simulink model "PID_Tuning"  (R2016b)
settings: Solver=ode45  StartTime=0.0  StopTime=10.0  RelTol=1e-3  EnableMultiTasking=on
values from neighbouring files (symbols this model uses):
  dm = 3.8E-6    (= 3.8e-06)    [param.m]    (also in param_2.m)
  eps_dm = 1    [param.m]    (also in param_2.m)
  eps_Jeq = 1    [param.m]    (also in param_2.m)
  Jeq = Jm + (J1+J2)/(n^2)    (= 3.6746e-05)    [param.m]    (also in param_2.m)
  Kemf = 1/(137*2*pi/60)    (= 0.0697028947848)    [param.m]    (also in param_2.m)
  Km = 69.7E-3    (= 0.0697)    [param.m]    (also in param_2.m)
  n = 1    [param.m]    (also in param_2.m)
  R = 112    [param.m]    (also in param_2.m)
  Ts = 1e-2    (= 0.01)    [param.m]    (also in param_2.m = 0.001)
libraries: simulink x1
settings Model: Creator=diegogm  LastModifiedBy=diego
settings DataIOCC: LimitDataPoints=on
settings OptimizationCC: LifeSpan=inf
settings DebuggingCC: AllowSymbolicDim=off  SFUnexpectedBacktrackingDiag=warning  SFNoUnconditionalDefaultTransitionDiag=warning  SFExecutionAtInitializationDiag=none
settings ModelReferenceCC: PropagateSignalLabelsOutOfModel=off
settings GRTTargetCC: TargetLangStandard=C89/C90 (ANSI)
settings ConfigComp: CovMetricSettings=dw  CovHtmlReporting=on  CovSaveCumulativeToWorkspaceVar=on  CovSaveSingleToWorkspaceVar=on  CovExternalEMLEnable=off

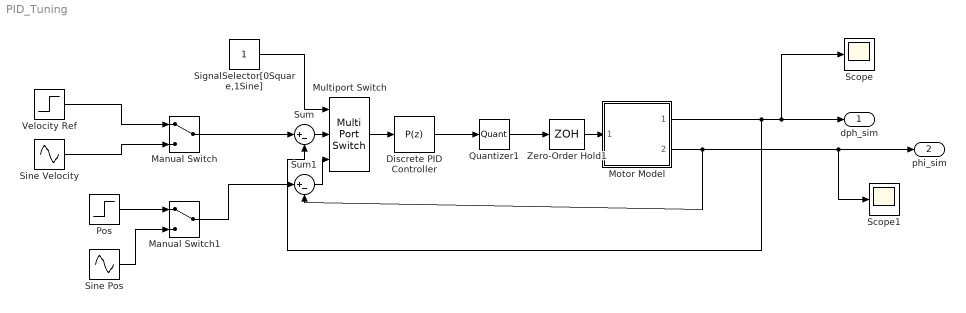
== system PID_Tuning ==
  Discrete PID Controller : simulink/Continuous/PID Controller  Controller=P  TimeDomain=Discrete-time  SampleTime=Ts  IntegratorMethod=Forward Euler  FilterMethod=Forward Euler  Form=Parallel  UseFilter=on  ControllerParametersSource=internal  P=1  I=1  D=1  N=1  InitialConditionSource=internal  InitialConditionForIntegrator=0  InitialConditionForFilter=0  ExternalReset=none  LimitOutput=off  UpperSaturationLimit=inf  LowerSaturationLimit=-inf  LinearizeAsGain=off  AntiWindupMode=none  Kb=1  TrackingMode=off  Kt=1  PParamMin=[]  PParamMax=[]  IParamMin=[]  IParamMax=[]  DParamMin=[]  DParamMax=[]  NParamMin=[]  NParamMax=[]  KbParamMin=[]  KbParamMax=[]  KtParamMin=[]  KtParamMax=[]  POutMin=[]  POutMax=[]  IOutMin=[]  IOutMax=[]  DOutMin=[]  DOutMax=[]  NOutMin=[]  NOutMax=[]  KbOutMin=[]  KbOutMax=[]  KtOutMin=[]  KtOutMax=[]  IntegratorOutMin=[]  IntegratorOutMax=[]  FilterOutMin=[]  FilterOutMax=[]  SumOutMin=[]  SumOutMax=[]  SumI1OutMin=[]  SumI1OutMax=[]  SumI2OutMin=[]  SumI2OutMax=[]  SumI3OutMin=[]  SumI3OutMax=[]  SumDOutMin=[]  SumDOutMax=[]  SaturationOutMin=[]  SaturationOutMax=[]  IntegratorContinuousStateAttributes=''  IntegratorStateMustResolveToSignalObject=off  IntegratorRTWStateStorageClass=Auto  FilterContinuousStateAttributes=''  FilterStateMustResolveToSignalObject=off  FilterRTWStateStorageClass=Auto  DifferentiatorICPrevScaledInput=0  DifferentiatorOutMin=[]  DifferentiatorOutMax=[]
  Manual Switch : ManualSwitch
  Manual Switch1 : ManualSwitch
  Motor Model : Subsystem
  Multiport Switch : MultiPortSwitch  Inputs=2
  Pos : Step  Time=0  SampleTime=0
  Quantizer1 : Quantizer  QuantizationInterval=Pulses  LinearizeAsGain=off  SampleTime=Ts
  Scope : Scope
  Scope1 : Scope
  SignalSelector[0Square,1Sine] : Constant
  Sine Pos : Sin  SampleTime=0
  Sine Velocity : Sin  SampleTime=0
  Sum : Sum  Inputs=|+-
  Sum1 : Sum  Inputs=|+-
  "Velocity Ref " : Step  Time=0  SampleTime=0
  Zero-Order Hold1 : ZeroOrderHold  SampleTime=Ts
  dph_sim : Outport
  phi_sim : Outport  Port=2
  wires:
  Motor Model/2(phi_sim) -> Sum1/2, Scope1/1, phi_sim/1
  SignalSelector[0Square,1Sine]/1 -> Multiport Switch/1
  Sum/1 -> Multiport Switch/2
  Sum1/1 -> Multiport Switch/3
  Multiport Switch/1 -> Discrete PID Controller/1
  Motor Model/1(dph_sim) -> Sum/2, Scope/1, dph_sim/1
  Quantizer1/1 -> Zero-Order Hold1/1
  Discrete PID Controller/1 -> Quantizer1/1
  Zero-Order Hold1/1 -> Motor Model/1(Signal Input)
  Manual Switch/1 -> Sum/1
  "Velocity Ref "/1 -> Manual Switch/1
  Sine Velocity/1 -> Manual Switch/2
  Manual Switch1/1 -> Sum1/1
  Pos/1 -> Manual Switch1/1
  Sine Pos/1 -> Manual Switch1/2

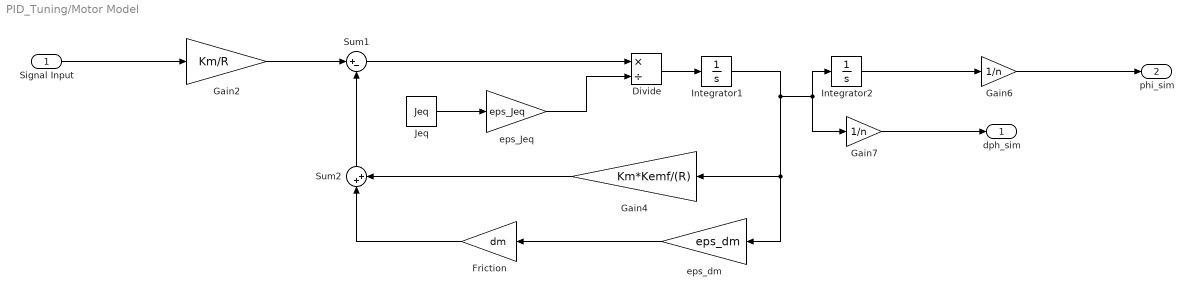
== system PID_Tuning/Motor Model ==
  Signal Input : Inport
  Divide : Product  Inputs=*/
  Friction : Gain  Gain=dm
  Gain2 : Gain  Gain=Km/R
  Gain4 : Gain  Gain=Km*Kemf/(R)
  Gain6 : Gain  Gain=1/n
  Gain7 : Gain  Gain=1/n
  Integrator1 : Integrator
  Integrator2 : Integrator
  Jeq : Constant  Value=Jeq
  Sum1 : Sum  Inputs=|+-
  Sum2 : Sum  Inputs=|++
  eps_Jeq : Gain  Gain=eps_Jeq
  eps_dm : Gain  Gain=eps_dm
  dph_sim : Outport
  phi_sim : Outport  Port=2
  wires:
  Integrator1/1 -> eps_dm/1, Gain4/1, Gain7/1, Integrator2/1
  Integrator2/1 -> Gain6/1
  Gain6/1 -> phi_sim/1
  Gain2/1 -> Sum1/1
  Divide/1 -> Integrator1/1
  Friction/1 -> Sum2/1
  Gain4/1 -> Sum2/2
  Sum2/1 -> Sum1/2
  Sum1/1 -> Divide/1
  Jeq/1 -> eps_Jeq/1
  eps_Jeq/1 -> Divide/2
  eps_dm/1 -> Friction/1
  Signal Input/1 -> Gain2/1
  Gain7/1 -> dph_sim/1
